simulink model "WM_Sim"  (R2013a)
settings: Solver=VariableStepDiscrete  StartTime=0.0  StopTime=WM.Sim.Time_length  RelTol=1e-3
InitFcn:
  | %if (matlab_sim)==false
  | 
  | %WM_Sim_config_smlnk_standalone;
  | 
  | %end
  | if isfield(WM.Sim,'BER_results')
  | WM.Sim = rmfield(WM.Sim,{'BER_results'});
  | end
  | if isfield(WM.Sim,'Uncoded_BER_results')
  | WM.Sim = rmfield(WM.Sim,{'Uncoded_BER_results'});
  | end
StopFcn:
  | if (matlab_sim)==false
  | WM.Sim.BER_results=BER_results_simout;
  | WM.Sim.Uncoded_BER_results=Uncoded_BER_results_simout;
  | %save_data_n_params(WM);
  | end
libraries: dspstat3 x15, dspmathops x8, dspsigops x3, dspsrcs4 x3, commdigbbndpm3 x3, commsink2 x2, commsynccomp2 x2, dspvision x2, commrandsrc2 x2, dspmtrx3 x2, commfilt2 x2, commchan3 x1
settings Model: Creator=leonardo  LastModifiedBy=leonardo
settings DataIOCC: SaveOutput=off  SignalLogging=off  DSMLogging=off  SaveTime=off
settings OptimizationCC: InlineParams=on  MemcpyThreshold=512
settings GRTTargetCC: CodeReplacementLibrary=C89/C90 (ANSI)

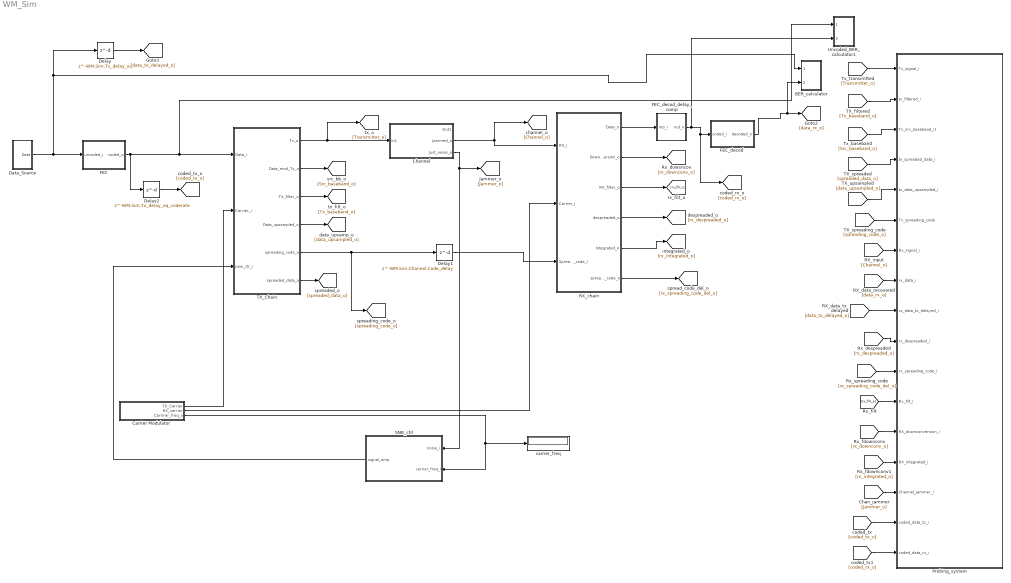
== system WM_Sim ==
  BER_calculator : Subsystem
  Carrier Modulator : Subsystem
  Channel : Subsystem
  Data_Source : Subsystem
  Delay : Delay  DelayLength=WM.Sim.Tx_delay_eq  InputProcessing=Columns as channels (frame based)
  Delay1 : Delay  DelayLength=WM.Sim.Channel.Code_delay  InputProcessing=Columns as channels (frame based)
  Delay2 : Delay  DelayLength=WM.Sim.Tx_delay_eq_coderate  InputProcessing=Columns as channels (frame based)
  FEC : Subsystem
  FEC_decod : Subsystem
  FEC_decod_delay_comp : Subsystem
  Probing_system : Subsystem
  RX_chain : Subsystem
  SNR_ctrl : Subsystem
  TX_Chain : Subsystem
  Uncoded_BER_calculator1 : Subsystem
  carrier_freq : Display
  wires:
  Carrier Modulator/1(TX_Carrier) -> TX_Chain/2(Carrier_i)
  TX_Chain/1(Tx_o) -> Channel/1(In1), [Transmitter_o]
  [Transmitter_o] -> Probing_system/1(Tx_signal_i)
  [Channel_o] -> Probing_system/7(Rx_signal_i)
  [data_tx_delayed_o] -> Probing_system/9(rx_data_tx_delayed_i)
  [data_rx_o] -> Probing_system/8(rx_data_i)
  TX_Chain/5(spreading_code_o) -> [spreading_code_o], Delay1/1
  Delay1/1 -> RX_chain/3(Spreading_code_i)
  TX_Chain/3(TX_filter_o) -> [Tx_baseband_o]
  [Tx_baseband_o] -> Probing_system/2(tx_filtered_i)
  TX_Chain/2(Data_mod_Tx_o) -> [Src_baseband_o]
  [Src_baseband_o] -> Probing_system/3(Tx_src_baseband_i1)
  TX_Chain/6(spreaded_data_o) -> [spreaded_data_o]
  [spreaded_data_o] -> Probing_system/4(tx_spreaded_data_i)
  [data_upsampled_o] -> Probing_system/5(tx_data_upsampled_i)
  RX_chain/3(RX_filter_o) -> [rx_filt_o]
  RX_chain/4(despreaded_o) -> [rx_despreaded_o]
  [rx_despreaded_o] -> Probing_system/10(rx_despreaded_i)
  [rx_spreading_code_del_o] -> Probing_system/11(rx_spreading_code_i)
  [spreading_code_o] -> Probing_system/6(Tx_spreading_code)
  [rx_filt_o] -> Probing_system/12(Rx_filt_i)
  RX_chain/2(Downconversion_o) -> [rx_downconv_o]
  [rx_downconv_o] -> Probing_system/13(RX_downconversion_i)
  RX_chain/5(Integrated_o) -> [rx_integrated_o]
  [rx_integrated_o] -> Probing_system/14(RX_integrated_i)
  Channel/3(Just_noise_o) -> [Jammer_o], SNR_ctrl/1(noise_i)
  SNR_ctrl/1(signal_amp) -> TX_Chain/3(pow_ctr_i)
  [Jammer_o] -> Probing_system/15(Channel_jammer_i)
  RX_chain/6(spreading_code_o) -> [rx_spreading_code_del_o]
  Carrier Modulator/3(Carrirer_freq_o) -> SNR_ctrl/2(carrier_freq_i), carrier_freq/1
  Data_Source/1(Data) -> FEC/1(uncoded_i), BER_calculator/1(Tx_delayed_data_i), Delay/1
  FEC/1(coded_o) -> TX_Chain/1(Data_i), Uncoded_BER_calculator1/1(Tx_delayed_data_i), Delay2/1
  Channel/2(Jammed_o) -> [Channel_o], RX_chain/1(RX_i)
  FEC_decod/1(decoded_o) -> BER_calculator/2(Rx_data_i), [data_rx_o]
  Carrier Modulator/2(RX_carrier) -> RX_chain/2(Carrier_i)
  TX_Chain/4(Data_upsampled_o) -> [data_upsampled_o]
  Delay/1 -> [data_tx_delayed_o]
  [coded_tx_o] -> Probing_system/16(coded_data_tx_i)
  Delay2/1 -> [coded_tx_o]
  [coded_rx_o] -> Probing_system/17(coded_data_rx_i)
  FEC_decod_delay_comp/1(out_o) -> Uncoded_BER_calculator1/2(Rx_data_i), [coded_rx_o], FEC_decod/1(coded_i)
  RX_chain/1(Data_o) -> FEC_decod_delay_comp/1(inp_i)

== system WM_Sim/BER_calculator ==
  Tx_delayed_data_i : Inport
  Rx_data_i : Inport  Port=2
  Display : Display
  Error Rate Calculation : commsink2/Error Rate Calculation  N=WM.Sim.Tx_delay_eq  st_delay=WM.Sim.Frame_len  cp_mode=Entire frame  subframe=[]  PMode=Port  WsName=ErrorVec  RsMode2=off  stop=off  numErr=100  maxBits=1e6
  To Workspace : ToWorkspace  VariableName=BER_results_simout  SampleTime=-1  SaveFormat=Timeseries
  wires:
  Rx_data_i/1 -> Error Rate Calculation/2
  Tx_delayed_data_i/1 -> Error Rate Calculation/1
  Error Rate Calculation/1 -> To Workspace/1, Display/1

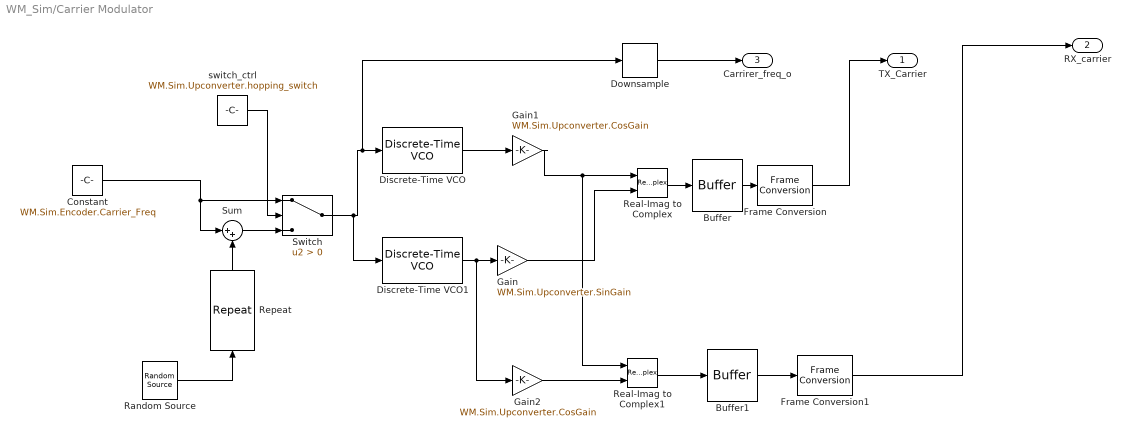
== system WM_Sim/Carrier Modulator ==
  Buffer : Buffer  N=int32(WM.Sim.Frame_len)  TreatMby1Signals=One channel
  Buffer1 : Buffer  N=int32(WM.Sim.Frame_len)  TreatMby1Signals=One channel
  Constant : Constant  Value=WM.Sim.Encoder.Carrier_Freq  VectorParams1D=off
  Discrete-Time VCO : commsynccomp2/Discrete-Time VCO  Ac=1  Fc=0  Kc=1  Ph=0  ts=WM.Sim.SampleTimes.Tchannel
  Discrete-Time VCO1 : commsynccomp2/Discrete-Time VCO  Ac=1  Fc=0  Kc=1  Ph=pi/4  ts=WM.Sim.SampleTimes.Tchannel
  Downsample : dspsigops/Downsample  N=int32(WM.Sim.Frame_len)  phase=0  InputProcessing=Columns as channels (frame based)  RateOptions=Allow multirate processing  smode=Allow multirate  fmode=Maintain input frame size  ic=0
  Frame Conversion : FrameConversion
  Frame Conversion1 : FrameConversion
  Gain : Gain  Gain=WM.Sim.Upconverter.SinGain
  Gain1 : Gain  Gain=WM.Sim.Upconverter.CosGain
  Gain2 : Gain  Gain=WM.Sim.Upconverter.CosGain
  Random Source : dspsrcs4/Random Source  SrcType=Uniform  NormMethod=Ziggurat  CltLength=12  MinVal=-WM.Sim.Upconverter.hopping_band/2  MaxVal=+WM.Sim.Upconverter.hopping_band/2  MeanVal=0  VarVal=1  RepMode=Specify seed  rawSeed=WM.Sim.Upconverter.Seed_hopping  IsInherit=off  SampMode=Discrete  SampTime=WM.Sim.SampleTimes.Tchannel*WM.Sim.Upconverter.hopping_div_vact  SampFrame=1  DataType=Double  OutComplex=Real
  Real-Imag to Complex : RealImagToComplex
  Real-Imag to Complex1 : RealImagToComplex
  Repeat : dspsigops/Repeat  N=WM.Sim.Upconverter.hopping_div_vact  InputProcessing=Columns as channels (frame based)  RateOptions=Allow multirate processing  ic=0  mode=Unused parameter value
  Sum : Sum  Inputs=|++
  Switch : Switch  Criteria=u2 > Threshold
  switch_ctrl : Constant  Value=WM.Sim.Upconverter.hopping_switch
  TX_Carrier : Outport
  RX_carrier : Outport  Port=2
  Carrirer_freq_o : Outport  Port=3
  wires:
  Buffer/1 -> Frame Conversion/1
  Gain/1 -> Real-Imag to Complex/2
  Buffer1/1 -> Frame Conversion1/1
  Constant/1 -> Switch/1, Sum/1
  Frame Conversion/1 -> TX_Carrier/1
  Discrete-Time VCO1/1 -> Gain2/1, Gain/1
  Real-Imag to Complex1/1 -> Buffer1/1
  Frame Conversion1/1 -> RX_carrier/1
  Discrete-Time VCO/1 -> Gain1/1
  Gain1/1 -> Real-Imag to Complex1/1, Real-Imag to Complex/1
  Gain2/1 -> Real-Imag to Complex1/2
  Real-Imag to Complex/1 -> Buffer/1
  Random Source/1 -> Repeat/1
  Sum/1 -> Switch/3
  Switch/1 -> Discrete-Time VCO1/1, Downsample/1, Discrete-Time VCO/1
  switch_ctrl/1 -> Switch/2
  Repeat/1 -> Sum/2
  Downsample/1 -> Carrirer_freq_o/1

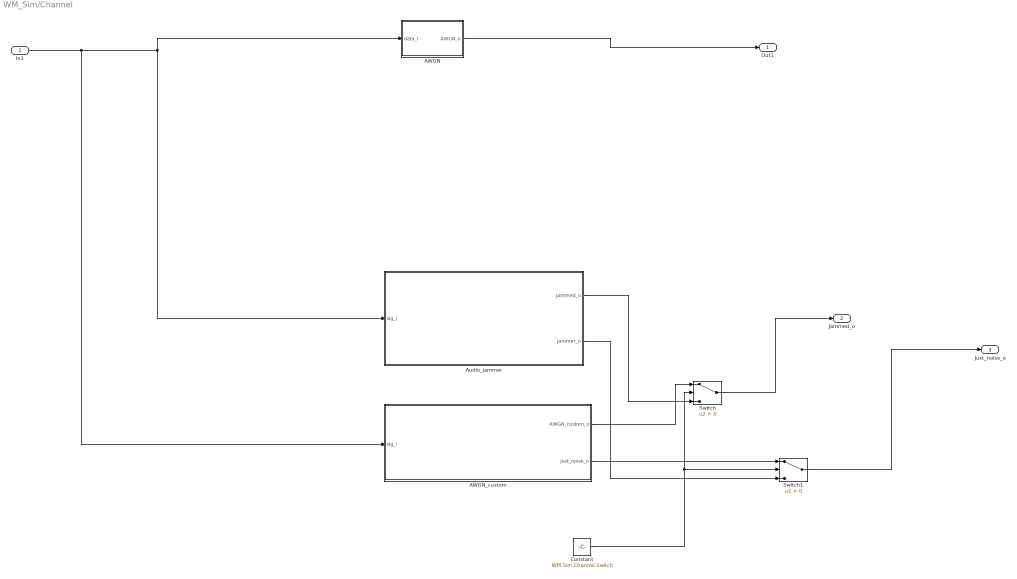
== system WM_Sim/Channel ==
  In1 : Inport
  AWGN : Subsystem
  AWGN_custom : Subsystem
  Audio_jammer : Subsystem
  Constant : Constant  Value=WM.Sim.Channel.Switch  SampleTime=WM.Sim.Frame_len/WM.Sim.Fs_audio
  Switch : Switch  Criteria=u2 > Threshold
  Switch1 : Switch  Criteria=u2 > Threshold
  Out1 : Outport
  Jammed_o : Outport  Port=2
  Just_noise_o : Outport  Port=3
  wires:
  In1/1 -> AWGN_custom/1(sig_i), Audio_jammer/1(sig_i), AWGN/1(data_i)
  AWGN/1(AWGN_o) -> Out1/1
  Constant/1 -> Switch1/2, Switch/2
  AWGN_custom/1(AWGN_custom_o) -> Switch/1
  Switch/1 -> Jammed_o/1
  Switch1/1 -> Just_noise_o/1
  AWGN_custom/2(just_noise_o) -> Switch1/1
  Audio_jammer/1(Jammed_o) -> Switch/3
  Audio_jammer/2(jammer_o) -> Switch1/3

== system WM_Sim/Data_Source ==
  Buffer : Buffer  N=WM.Sim.Frame_len  TreatMby1Signals=One channel
  Constant : Constant  VectorParams1D=off  SampleTime=WM.Sim.SampleTimes.Tsource  FramePeriod=WM.Sim.SampleTimes.Tsource
  Constant1 : Constant  Value=WM.Sim.Encoder.Source.Switch  VectorParams1D=off  FramePeriod=WM.Sim.SampleTimes.Tspreader
  Frame Conversion : FrameConversion
  Random Integer Generator : commrandsrc2/Random Integer Generator  mul=WM.Sim.order_M  seed=WM.Sim.seed_rand_msg  Ts=WM.Sim.SampleTimes.Tsource  frameBased=on  sampPerFrame=WM.Sim.Frame_len  orient=off  outDataType=double
  Switch : Switch  Criteria=u2 > Threshold
  Data : Outport
  wires:
  Random Integer Generator/1 -> Switch/1
  Constant/1 -> Buffer/1
  Buffer/1 -> Frame Conversion/1
  Frame Conversion/1 -> Switch/3
  Constant1/1 -> Switch/2
  Switch/1 -> Data/1

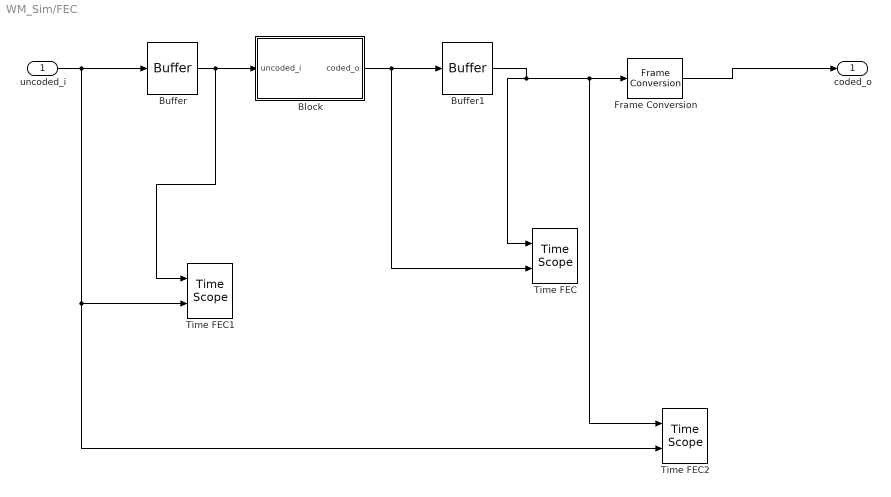
== system WM_Sim/FEC ==
  uncoded_i : Inport
  Block : Subsystem
  Buffer : Buffer  N=WM.Sim.Message_length  TreatMby1Signals=One channel
  Buffer1 : Buffer  N=WM.Sim.Frame_len  TreatMby1Signals=One channel
  Frame Conversion : FrameConversion
  Time FEC : TimeScope  NumInputPorts=2  DefaultConfigurationName=spbscopes.TimeScopeBlockCfg
      settings: CopyFcn=scopeextensions.ScopeBlock.callback(gcbh, 'onBlockCopy', gcbh);  DeleteFcn=scopeextensions.ScopeBlock.callback(gcbh, 'onBlockDelete');  PreSaveFcn=scopeextensions.ScopeBlock.callback(gcbh, 'onModelSave');  NameChangeFcn=scopeextensions.ScopeBlock.callback(gcbh, 'onBlockRename');  CloseFcn=scopeextensions.ScopeBlock.callback(gcbh, 'onBlockClose');  PreDeleteFcn=scopeextensions.ScopeBlock.callback(gcbh, 'onBlockPreDelete');
  Time FEC1 : TimeScope  NumInputPorts=2  DefaultConfigurationName=spbscopes.TimeScopeBlockCfg
      settings: CopyFcn=scopeextensions.ScopeBlock.callback(gcbh, 'onBlockCopy', gcbh);  DeleteFcn=scopeextensions.ScopeBlock.callback(gcbh, 'onBlockDelete');  PreSaveFcn=scopeextensions.ScopeBlock.callback(gcbh, 'onModelSave');  NameChangeFcn=scopeextensions.ScopeBlock.callback(gcbh, 'onBlockRename');  CloseFcn=scopeextensions.ScopeBlock.callback(gcbh, 'onBlockClose');  PreDeleteFcn=scopeextensions.ScopeBlock.callback(gcbh, 'onBlockPreDelete');
  Time FEC2 : TimeScope  NumInputPorts=2  DefaultConfigurationName=spbscopes.TimeScopeBlockCfg
      settings: CopyFcn=scopeextensions.ScopeBlock.callback(gcbh, 'onBlockCopy', gcbh);  DeleteFcn=scopeextensions.ScopeBlock.callback(gcbh, 'onBlockDelete');  PreSaveFcn=scopeextensions.ScopeBlock.callback(gcbh, 'onModelSave');  NameChangeFcn=scopeextensions.ScopeBlock.callback(gcbh, 'onBlockRename');  CloseFcn=scopeextensions.ScopeBlock.callback(gcbh, 'onBlockClose');  PreDeleteFcn=scopeextensions.ScopeBlock.callback(gcbh, 'onBlockPreDelete');
  coded_o : Outport
  wires:
  uncoded_i/1 -> Time FEC2/2, Time FEC1/2, Buffer/1
  Frame Conversion/1 -> coded_o/1
  Block/1(coded_o) -> Time FEC/2, Buffer1/1
  Buffer1/1 -> Time FEC/1, Time FEC2/1, Frame Conversion/1
  Buffer/1 -> Time FEC1/1, Block/1(uncoded_i)

== system WM_Sim/FEC_decod ==
  coded_i : Inport
  Block : Subsystem
  Buffer : Buffer  N=WM.Sim.Codeword_length  TreatMby1Signals=One channel
  Frame Conversion : FrameConversion
  Time FEC_decod : TimeScope  NumInputPorts=2  DefaultConfigurationName=spbscopes.TimeScopeBlockCfg
      settings: CopyFcn=scopeextensions.ScopeBlock.callback(gcbh, 'onBlockCopy', gcbh);  DeleteFcn=scopeextensions.ScopeBlock.callback(gcbh, 'onBlockDelete');  PreSaveFcn=scopeextensions.ScopeBlock.callback(gcbh, 'onModelSave');  NameChangeFcn=scopeextensions.ScopeBlock.callback(gcbh, 'onBlockRename');  CloseFcn=scopeextensions.ScopeBlock.callback(gcbh, 'onBlockClose');  PreDeleteFcn=scopeextensions.ScopeBlock.callback(gcbh, 'onBlockPreDelete');
  Time FEC_decod1 : TimeScope  NumInputPorts=2  DefaultConfigurationName=spbscopes.TimeScopeBlockCfg
      settings: CopyFcn=scopeextensions.ScopeBlock.callback(gcbh, 'onBlockCopy', gcbh);  DeleteFcn=scopeextensions.ScopeBlock.callback(gcbh, 'onBlockDelete');  PreSaveFcn=scopeextensions.ScopeBlock.callback(gcbh, 'onModelSave');  NameChangeFcn=scopeextensions.ScopeBlock.callback(gcbh, 'onBlockRename');  CloseFcn=scopeextensions.ScopeBlock.callback(gcbh, 'onBlockClose');  PreDeleteFcn=scopeextensions.ScopeBlock.callback(gcbh, 'onBlockPreDelete');
  Unbuff : Subsystem
  decoded_o : Outport
  wires:
  coded_i/1 -> Time FEC_decod1/2, Buffer/1
  Frame Conversion/1 -> decoded_o/1
  Buffer/1 -> Time FEC_decod1/1, Block/1(coded_i)
  Block/1(decoded_o) -> Time FEC_decod/2, Unbuff/1(buffered_i)
  Unbuff/1(unbuffered_o) -> Time FEC_decod/1, Frame Conversion/1

== system WM_Sim/FEC_decod_delay_comp ==
  inp_i : Inport
  out_o : Outport
  wires:
  inp_i/1 -> out_o/1

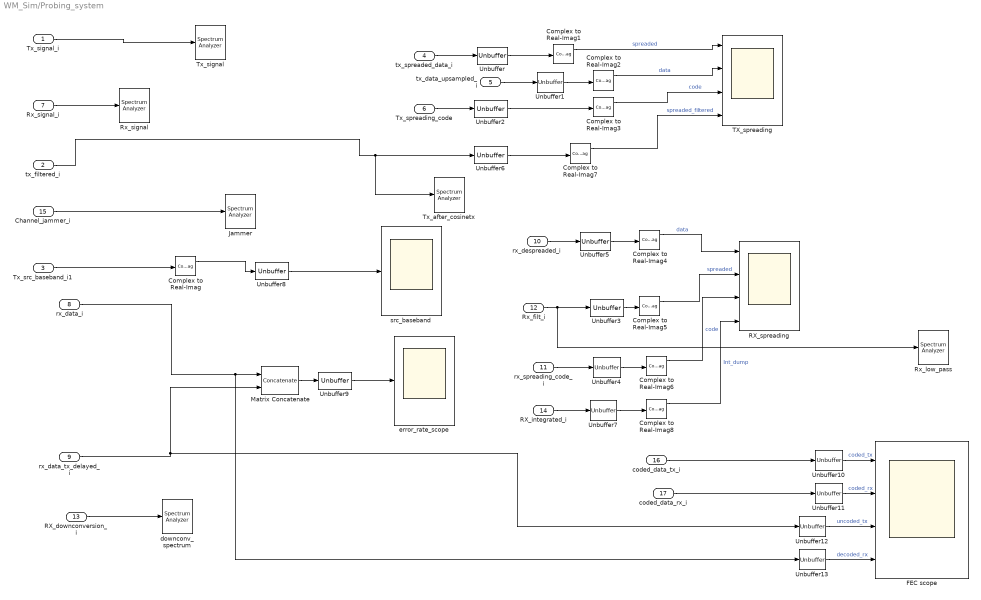
== system WM_Sim/Probing_system ==
  Tx_signal_i : Inport
  tx_filtered_i : Inport  Port=2
  Tx_src_baseband_i1 : Inport  Port=3
  tx_spreaded_data_i : Inport  Port=4
  tx_data_upsampled_i : Inport  Port=5
  Tx_spreading_code : Inport  Port=6
  Rx_signal_i : Inport  Port=7
  rx_data_i : Inport  Port=8
  rx_data_tx_delayed_i : Inport  Port=9
  rx_despreaded_i : Inport  Port=10
  rx_spreading_code_i : Inport  Port=11
  Rx_filt_i : Inport  Port=12
  RX_downconversion_i : Inport  Port=13
  RX_integrated_i : Inport  Port=14
  Channel_jammer_i : Inport  Port=15
  coded_data_tx_i : Inport  Port=16
  coded_data_rx_i : Inport  Port=17
  Complex to Real-Imag{,1..8} (9 alike) : ComplexToRealImag
  FEC scope : Scope  NumInputPorts=4
      settings: YMin=-5~-5~-5~-5  YMax=5~5~5~5  SaveName=ScopeData6
  Jammer : SpectrumAnalyzer
      settings: CopyFcn=scopeextensions.ScopeBlock.callback(gcbh, 'onBlockCopy', gcbh);  DeleteFcn=scopeextensions.ScopeBlock.callback(gcbh, 'onBlockDelete');  PreSaveFcn=scopeextensions.ScopeBlock.callback(gcbh, 'onModelSave');  NameChangeFcn=scopeextensions.ScopeBlock.callback(gcbh, 'onBlockRename');  CloseFcn=scopeextensions.ScopeBlock.callback(gcbh, 'onBlockClose');  PreDeleteFcn=scopeextensions.ScopeBlock.callback(gcbh, 'onBlockPreDelete');
  Matrix Concatenate : Concatenate  Mode=Multidimensional array  ConcatenateDimension=2
  RX_spreading : Scope  NumInputPorts=4
      settings: YMin=-0.0225~-0.025~-1~-1000  YMax=0.02~0.025~1~1750  SaveName=ScopeData3  MaxDataPoints=WM.Sim.Probe_system.RX_spreading.data_history_len
  Rx_low_pass : SpectrumAnalyzer
      settings: CopyFcn=scopeextensions.ScopeBlock.callback(gcbh, 'onBlockCopy', gcbh);  DeleteFcn=scopeextensions.ScopeBlock.callback(gcbh, 'onBlockDelete');  PreSaveFcn=scopeextensions.ScopeBlock.callback(gcbh, 'onModelSave');  NameChangeFcn=scopeextensions.ScopeBlock.callback(gcbh, 'onBlockRename');  CloseFcn=scopeextensions.ScopeBlock.callback(gcbh, 'onBlockClose');  PreDeleteFcn=scopeextensions.ScopeBlock.callback(gcbh, 'onBlockPreDelete');
  Rx_signal : SpectrumAnalyzer
      settings: CopyFcn=scopeextensions.ScopeBlock.callback(gcbh, 'onBlockCopy', gcbh);  DeleteFcn=scopeextensions.ScopeBlock.callback(gcbh, 'onBlockDelete');  PreSaveFcn=scopeextensions.ScopeBlock.callback(gcbh, 'onModelSave');  NameChangeFcn=scopeextensions.ScopeBlock.callback(gcbh, 'onBlockRename');  CloseFcn=scopeextensions.ScopeBlock.callback(gcbh, 'onBlockClose');  PreDeleteFcn=scopeextensions.ScopeBlock.callback(gcbh, 'onBlockPreDelete');
  TX_spreading : Scope  NumInputPorts=4
      settings: YMin=-5~-5~-5~-5  YMax=5~5~5~5  SaveName=ScopeData2
  Tx_after_cosinetx : SpectrumAnalyzer
      settings: CopyFcn=scopeextensions.ScopeBlock.callback(gcbh, 'onBlockCopy', gcbh);  DeleteFcn=scopeextensions.ScopeBlock.callback(gcbh, 'onBlockDelete');  PreSaveFcn=scopeextensions.ScopeBlock.callback(gcbh, 'onModelSave');  NameChangeFcn=scopeextensions.ScopeBlock.callback(gcbh, 'onBlockRename');  CloseFcn=scopeextensions.ScopeBlock.callback(gcbh, 'onBlockClose');  PreDeleteFcn=scopeextensions.ScopeBlock.callback(gcbh, 'onBlockPreDelete');
  Tx_signal : SpectrumAnalyzer
      settings: CopyFcn=scopeextensions.ScopeBlock.callback(gcbh, 'onBlockCopy', gcbh);  DeleteFcn=scopeextensions.ScopeBlock.callback(gcbh, 'onBlockDelete');  PreSaveFcn=scopeextensions.ScopeBlock.callback(gcbh, 'onModelSave');  NameChangeFcn=scopeextensions.ScopeBlock.callback(gcbh, 'onBlockRename');  CloseFcn=scopeextensions.ScopeBlock.callback(gcbh, 'onBlockClose');  PreDeleteFcn=scopeextensions.ScopeBlock.callback(gcbh, 'onBlockPreDelete');
  Unbuffer{,1..13} (14 alike) : Unbuffer  SampleBasedProcessing=Same as frame based
  downconv_spectrum : SpectrumAnalyzer
      settings: CopyFcn=scopeextensions.ScopeBlock.callback(gcbh, 'onBlockCopy', gcbh);  DeleteFcn=scopeextensions.ScopeBlock.callback(gcbh, 'onBlockDelete');  PreSaveFcn=scopeextensions.ScopeBlock.callback(gcbh, 'onModelSave');  NameChangeFcn=scopeextensions.ScopeBlock.callback(gcbh, 'onBlockRename');  CloseFcn=scopeextensions.ScopeBlock.callback(gcbh, 'onBlockClose');  PreDeleteFcn=scopeextensions.ScopeBlock.callback(gcbh, 'onBlockPreDelete');
  error_rate_scope : Scope
  src_baseband : Scope
  wires:
  Rx_signal_i/1 -> Rx_signal/1
  Matrix Concatenate/1 -> Unbuffer9/1
  rx_data_tx_delayed_i/1 -> Unbuffer12/1, Matrix Concatenate/2
  rx_data_i/1 -> Unbuffer13/1, Matrix Concatenate/1
  tx_filtered_i/1 -> Tx_after_cosinetx/1, Unbuffer6/1
  Tx_src_baseband_i1/1 -> Complex to Real-Imag/1
  Complex to Real-Imag/1 -> Unbuffer8/1
  tx_data_upsampled_i/1 -> Unbuffer1/1
  tx_spreaded_data_i/1 -> Unbuffer/1
  Tx_spreading_code/1 -> Unbuffer2/1
  Complex to Real-Imag1/1 -> TX_spreading/1  "spreaded"
  Unbuffer/1 -> Complex to Real-Imag1/1
  Unbuffer1/1 -> Complex to Real-Imag2/1
  Unbuffer2/1 -> Complex to Real-Imag3/1
  Complex to Real-Imag2/1 -> TX_spreading/2  "data"
  Complex to Real-Imag3/1 -> TX_spreading/3  "code"
  rx_despreaded_i/1 -> Unbuffer5/1
  rx_spreading_code_i/1 -> Unbuffer4/1
  Rx_filt_i/1 -> Rx_low_pass/1, Unbuffer3/1
  Unbuffer5/1 -> Complex to Real-Imag4/1
  Unbuffer3/1 -> Complex to Real-Imag5/1
  Unbuffer4/1 -> Complex to Real-Imag6/1
  Complex to Real-Imag4/1 -> RX_spreading/1  "data"
  Complex to Real-Imag5/1 -> RX_spreading/2  "spreaded"
  Complex to Real-Imag6/1 -> RX_spreading/3  "code"
  Complex to Real-Imag7/1 -> TX_spreading/4  "spreaded_filtered"
  Unbuffer6/1 -> Complex to Real-Imag7/1
  RX_integrated_i/1 -> Unbuffer7/1
  Unbuffer7/1 -> Complex to Real-Imag8/1
  Complex to Real-Imag8/1 -> RX_spreading/4  "Int_dump"
  Channel_jammer_i/1 -> Jammer/1
  Tx_signal_i/1 -> Tx_signal/1
  RX_downconversion_i/1 -> downconv_spectrum/1
  Unbuffer8/1 -> src_baseband/1
  Unbuffer9/1 -> error_rate_scope/1
  Unbuffer12/1 -> FEC scope/3  "uncoded_tx"
  Unbuffer10/1 -> FEC scope/1  "coded_tx"
  Unbuffer13/1 -> FEC scope/4  "decoded_rx"
  Unbuffer11/1 -> FEC scope/2  "coded_rx"
  coded_data_tx_i/1 -> Unbuffer10/1
  coded_data_rx_i/1 -> Unbuffer11/1

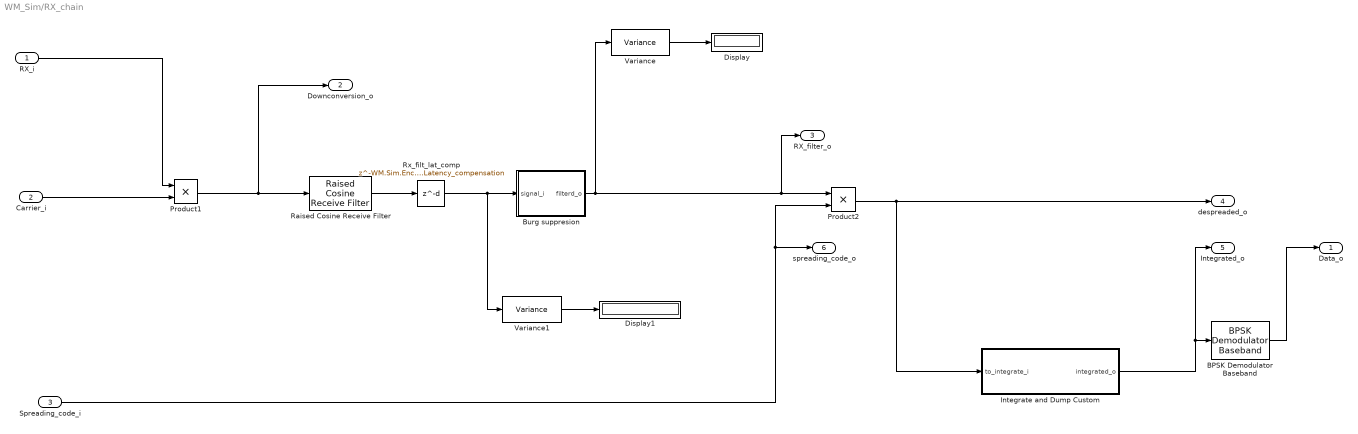
== system WM_Sim/RX_chain ==
  RX_i : Inport
  Carrier_i : Inport  Port=2
  Spreading_code_i : Inport  Port=3
  BPSK Demodulator Baseband : commdigbbndpm3/BPSK Demodulator Baseband  Ph=0  DecType=Hard decision  VarSource=Dialog  Variance=1  outDtype=Inherit via internal rule  derotateFactorWordLen=16
  Burg suppresion : Subsystem
  Display : Display
  Display1 : Display
  Integrate and Dump Custom : Subsystem
  Product1 : Product
  Product2 : Product
  Raised Cosine Receive Filter : commfilt2/Raised Cosine Receive Filter  filtType=Normal  N=WM.Sim.Encoder.TxFilter.OversamplingFactor  D=(2*(WM.Sim.Encoder.TxFilter.GroupDelay))/2  R=WM.Sim.Encoder.TxFilter.RollOffFactor  sampMode=Mute  saveAsFlag=0  rateMode=Downsampling  downFactor=WM.Sim.Encoder.TxFilter.OversamplingFactor  downOffset=0  framing=Allow multirate processing  InputProcessing=Columns as channels (frame based)  checkGain=User-specified  filterGain=1  checkCoeff=on  variableName=hRxFilt  launchFVT=off  roundingMode=Floor  overflowMode=off
  Rx_filt_lat_comp : Delay  DelayLength=WM.Sim.Encoder.TxFilter.Latency_compensation  InputProcessing=Columns as channels (frame based)
  Variance : dspstat3/Variance  run=on  reset_popup=None  InputProcessing=Columns as channels (frame based)  directionMode=Each column  dimension=1  treatSBRowAsCol=on  roiEnable=off  roiType=Rectangles  roiPortion=Entire ROI  roiOutput=Individual statistics for each ROI  roiFlag=off  roundingMode=Floor  overflowMode=off
  Variance1 : dspstat3/Variance  run=on  reset_popup=None  InputProcessing=Columns as channels (frame based)  directionMode=Each column  dimension=1  treatSBRowAsCol=on  roiEnable=off  roiType=Rectangles  roiPortion=Entire ROI  roiOutput=Individual statistics for each ROI  roiFlag=off  roundingMode=Floor  overflowMode=off
  Data_o : Outport
  Downconversion_o : Outport  Port=2
  RX_filter_o : Outport  Port=3
  despreaded_o : Outport  Port=4
  Integrated_o : Outport  Port=5
  spreading_code_o : Outport  Port=6
  wires:
  BPSK Demodulator Baseband/1 -> Data_o/1
  Product1/1 -> Raised Cosine Receive Filter/1, Downconversion_o/1
  Raised Cosine Receive Filter/1 -> Rx_filt_lat_comp/1
  RX_i/1 -> Product1/1
  Carrier_i/1 -> Product1/2
  Integrate and Dump Custom/1(integrated_o) -> Integrated_o/1, BPSK Demodulator Baseband/1
  Product2/1 -> Integrate and Dump Custom/1(to_integrate_i), despreaded_o/1
  Burg suppresion/1(filterd_o) -> Variance/1, RX_filter_o/1, Product2/1
  Rx_filt_lat_comp/1 -> Burg suppresion/1(signal_i), Variance1/1
  Spreading_code_i/1 -> spreading_code_o/1, Product2/2
  Variance/1 -> Display/1
  Variance1/1 -> Display1/1

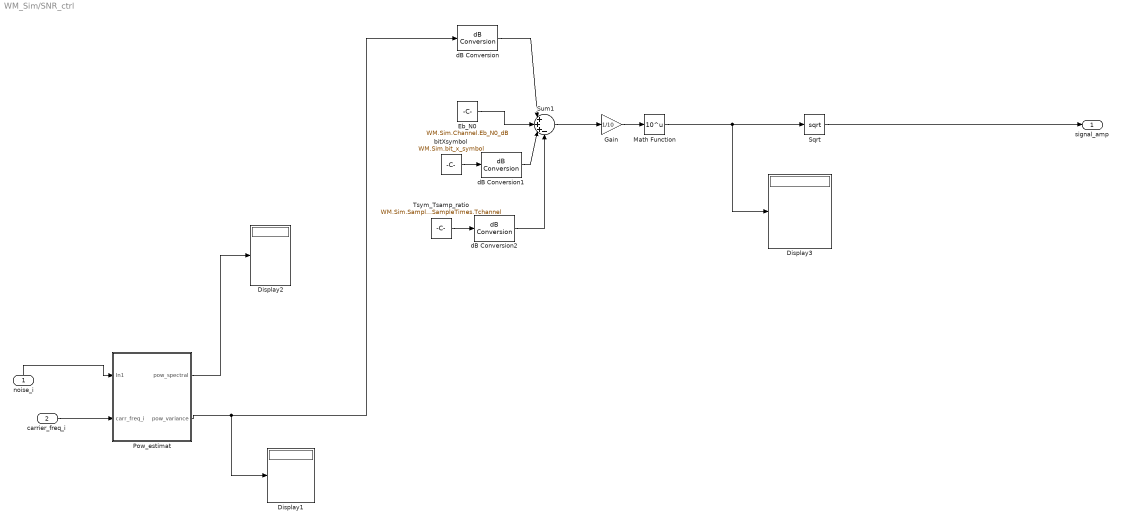
== system WM_Sim/SNR_ctrl ==
  noise_i : Inport
  carrier_freq_i : Inport  Port=2
  Display1 : Display
  Display2 : Display
  Display3 : Display
  Eb_N0 : Constant  Value=WM.Sim.Channel.Eb_N0_dB
  Gain : Gain  Gain=1/10
  Math Function : Math  Operator=10^u  SaturateOnIntegerOverflow=on
  Pow_estimat : Subsystem
  Sqrt : Sqrt  SaturateOnIntegerOverflow=on
  Sum1 : Sum  Inputs=|+++-
  Tsym_Tsamp_ratio : Constant  Value=WM.Sim.SampleTimes.Tcoded/WM.Sim.SampleTimes.Tchannel
      settings: SamplingMode=Frame based
  bitXsymbol : Constant  Value=WM.Sim.bit_x_symbol
  dB Conversion : dspmathops/dB Conversion  dBtype=dB  intype=Power  R=1  fuzz=off
  dB Conversion1 : dspmathops/dB Conversion  dBtype=dB  intype=Power  R=1  fuzz=off
  dB Conversion2 : dspmathops/dB Conversion  dBtype=dB  intype=Power  R=1  fuzz=off
  signal_amp : Outport
  wires:
  Sum1/1 -> Gain/1
  Eb_N0/1 -> Sum1/2
  Tsym_Tsamp_ratio/1 -> dB Conversion2/1
  dB Conversion/1 -> Sum1/1
  dB Conversion2/1 -> Sum1/4
  bitXsymbol/1 -> dB Conversion1/1
  dB Conversion1/1 -> Sum1/3
  Gain/1 -> Math Function/1
  Math Function/1 -> Display3/1, Sqrt/1
  Sqrt/1 -> signal_amp/1
  Pow_estimat/2(pow_variance) -> Display1/1, dB Conversion/1
  noise_i/1 -> Pow_estimat/1(In1)
  Pow_estimat/1(pow_spectral) -> Display2/1
  carrier_freq_i/1 -> Pow_estimat/2(carr_freq_i)

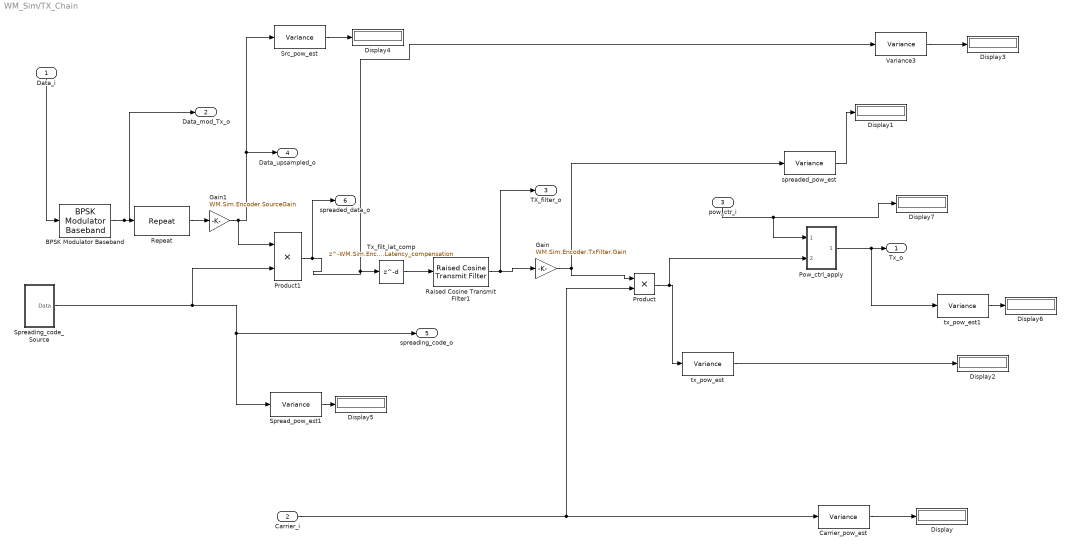
== system WM_Sim/TX_Chain ==
  Data_i : Inport
  Carrier_i : Inport  Port=2
  pow_ctr_i : Inport  Port=3
  BPSK Modulator Baseband : commdigbbndpm3/BPSK Modulator Baseband  Ph=0  outDtype=double  outWordLen=16  outUDDataType=sfix(16)  outFracLenMode=Best precision  outFracLen=15
  Carrier_pow_est : dspstat3/Variance  run=on  reset_popup=None  InputProcessing=Columns as channels (frame based)  directionMode=Each column  dimension=1  treatSBRowAsCol=on  roiEnable=off  roiType=Rectangles  roiPortion=Entire ROI  roiOutput=Individual statistics for each ROI  roiFlag=off  roundingMode=Floor  overflowMode=off
  Display{,1..7} (8 alike) : Display
  Gain : Gain  Gain=WM.Sim.Encoder.TxFilter.Gain
  Gain1 : Gain  Gain=WM.Sim.Encoder.SourceGain
  Pow_ctrl_apply : Subsystem
  Product : Product
  Product1 : Product
  Raised Cosine Transmit Filter1 : commfilt2/Raised Cosine Transmit Filter  filtType=Normal  D=(2*(WM.Sim.Encoder.TxFilter.GroupDelay))/2  R=WM.Sim.Encoder.TxFilter.RollOffFactor  sampMode=Mute  saveAsFlag=0  N=WM.Sim.Encoder.TxFilter.OversamplingFactor  framing=Allow multirate processing  InputProcessing=Columns as channels (frame based)  checkGain=Normalized  filterGain=1  checkCoeff=off  variableName=rcTxFilt1  launchFVT=off  roundingMode=Floor  overflowMode=off
  Repeat : dspsigops/Repeat  N=WM.Sim.Encoder.SF  InputProcessing=Columns as channels (frame based)  RateOptions=Allow multirate processing  ic=0  mode=Unused parameter value
  Spread_pow_est1 : dspstat3/Variance  run=on  reset_popup=None  InputProcessing=Columns as channels (frame based)  directionMode=Each column  dimension=1  treatSBRowAsCol=on  roiEnable=off  roiType=Rectangles  roiPortion=Entire ROI  roiOutput=Individual statistics for each ROI  roiFlag=off  roundingMode=Floor  overflowMode=off
  Spreading_code_Source : Subsystem
  Src_pow_est : dspstat3/Variance  run=on  reset_popup=None  InputProcessing=Columns as channels (frame based)  directionMode=Each column  dimension=1  treatSBRowAsCol=on  roiEnable=off  roiType=Rectangles  roiPortion=Entire ROI  roiOutput=Individual statistics for each ROI  roiFlag=off  roundingMode=Floor  overflowMode=off
  Tx_filt_lat_comp : Delay  DelayLength=WM.Sim.Encoder.TxFilter.Latency_compensation  InputProcessing=Columns as channels (frame based)
  Variance3 : dspstat3/Variance  run=on  reset_popup=None  InputProcessing=Columns as channels (frame based)  directionMode=Each column  dimension=1  treatSBRowAsCol=on  roiEnable=off  roiType=Rectangles  roiPortion=Entire ROI  roiOutput=Individual statistics for each ROI  roiFlag=off  roundingMode=Floor  overflowMode=off
  spreaded_pow_est : dspstat3/Variance  run=on  reset_popup=None  InputProcessing=Columns as channels (frame based)  directionMode=Each column  dimension=1  treatSBRowAsCol=on  roiEnable=off  roiType=Rectangles  roiPortion=Entire ROI  roiOutput=Individual statistics for each ROI  roiFlag=off  roundingMode=Floor  overflowMode=off
  tx_pow_est : dspstat3/Variance  run=on  reset_popup=None  InputProcessing=Columns as channels (frame based)  directionMode=Each column  dimension=1  treatSBRowAsCol=on  roiEnable=off  roiType=Rectangles  roiPortion=Entire ROI  roiOutput=Individual statistics for each ROI  roiFlag=off  roundingMode=Floor  overflowMode=off
  tx_pow_est1 : dspstat3/Variance  run=on  reset_popup=None  InputProcessing=Columns as channels (frame based)  directionMode=Each column  dimension=1  treatSBRowAsCol=on  roiEnable=off  roiType=Rectangles  roiPortion=Entire ROI  roiOutput=Individual statistics for each ROI  roiFlag=off  roundingMode=Floor  overflowMode=off
  Tx_o : Outport
  Data_mod_Tx_o : Outport  Port=2
  TX_filter_o : Outport  Port=3
  Data_upsampled_o : Outport  Port=4
  spreading_code_o : Outport  Port=5
  spreaded_data_o : Outport  Port=6
  wires:
  Data_i/1 -> BPSK Modulator Baseband/1
  BPSK Modulator Baseband/1 -> Data_mod_Tx_o/1, Repeat/1
  Product/1 -> Pow_ctrl_apply/2(data_i), tx_pow_est/1
  Gain/1 -> Product/1, spreaded_pow_est/1
  Carrier_pow_est/1 -> Display/1
  spreaded_pow_est/1 -> Display1/1
  Spreading_code_Source/1(Data) -> Spread_pow_est1/1, spreading_code_o/1, Product1/2
  Repeat/1 -> Gain1/1
  tx_pow_est/1 -> Display2/1
  Variance3/1 -> Display3/1
  Gain1/1 -> Product1/1, Data_upsampled_o/1, Src_pow_est/1
  Src_pow_est/1 -> Display4/1
  Spread_pow_est1/1 -> Display5/1
  Product1/1 -> spreaded_data_o/1, Tx_filt_lat_comp/1, Variance3/1
  Pow_ctrl_apply/1(data_o) -> tx_pow_est1/1, Tx_o/1
  tx_pow_est1/1 -> Display6/1
  pow_ctr_i/1 -> Pow_ctrl_apply/1(ctrl_pow_i), Display7/1
  Carrier_i/1 -> Carrier_pow_est/1, Product/2
  Tx_filt_lat_comp/1 -> Raised Cosine Transmit Filter1/1
  Raised Cosine Transmit Filter1/1 -> TX_filter_o/1, Gain/1

== system WM_Sim/Uncoded_BER_calculator1 ==
  Tx_delayed_data_i : Inport
  Rx_data_i : Inport  Port=2
  Display : Display
  Error Rate Calculation : commsink2/Error Rate Calculation  N=WM.Sim.Tx_delay_eq_coderate  st_delay=WM.Sim.Frame_len  cp_mode=Entire frame  subframe=[]  PMode=Port  WsName=ErrorVec  RsMode2=off  stop=off  numErr=100  maxBits=1e6
  To Workspace : ToWorkspace  VariableName=Uncoded_BER_results_simout  SampleTime=-1  SaveFormat=Timeseries
  wires:
  Error Rate Calculation/1 -> Display/1, To Workspace/1
  Tx_delayed_data_i/1 -> Error Rate Calculation/1
  Rx_data_i/1 -> Error Rate Calculation/2

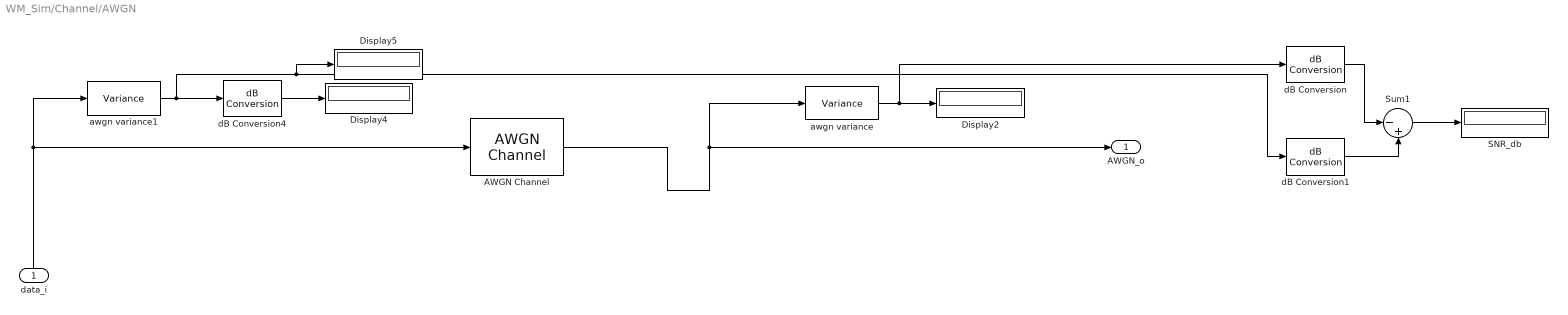
== system WM_Sim/Channel/AWGN ==
  data_i : Inport
  " awgn variance" : dspstat3/Variance  run=on  reset_popup=None  InputProcessing=Columns as channels (frame based)  directionMode=Each column  dimension=1  treatSBRowAsCol=on  roiEnable=off  roiType=Rectangles  roiPortion=Entire ROI  roiOutput=Individual statistics for each ROI  roiFlag=off  roundingMode=Floor  overflowMode=off
  " awgn variance1" : dspstat3/Variance  run=on  reset_popup=None  InputProcessing=Columns as channels (frame based)  directionMode=Each column  dimension=1  treatSBRowAsCol=on  roiEnable=off  roiType=Rectangles  roiPortion=Entire ROI  roiOutput=Individual statistics for each ROI  roiFlag=off  roundingMode=Floor  overflowMode=off
  AWGN Channel : commchan3/AWGN Channel  InputProcessing=Columns as channels (frame based)  seed=WM.Sim.Channel.AWGN_Custom.seed_noise_real  noiseMode="Signal to noise ratio  (Eb/No)"  EbNodB=WM.Sim.Channel.Eb_N0_dB  EsNodB=10  SNRdB=10  bitsPerSym=WM.Sim.bit_x_symbol  Ps=0.94  Tsym=WM.Sim.Encoder.Source_Ts  variance=1
  Display2 : Display
  Display4 : Display
  Display5 : Display
  SNR_db : Display
  Sum1 : Sum  Inputs=|-+
  dB Conversion : dspmathops/dB Conversion  dBtype=dB  intype=Power  R=1  fuzz=off
  dB Conversion1 : dspmathops/dB Conversion  dBtype=dB  intype=Power  R=1  fuzz=off
  dB Conversion4 : dspmathops/dB Conversion  dBtype=dB  intype=Power  R=1  fuzz=off
  AWGN_o : Outport
  wires:
  Sum1/1 -> SNR_db/1
  " awgn variance1"/1 -> Display5/1, dB Conversion1/1, dB Conversion4/1
  AWGN Channel/1 -> AWGN_o/1, " awgn variance"/1
  data_i/1 -> AWGN Channel/1, " awgn variance1"/1
  dB Conversion4/1 -> Display4/1
  dB Conversion1/1 -> Sum1/2
  dB Conversion/1 -> Sum1/1
  " awgn variance"/1 -> dB Conversion/1, Display2/1

== system WM_Sim/Channel/AWGN_custom ==
  sig_i : Inport
  AWGN Channel Custom : Subsystem
  Display1 : Display
  SNR_estimate : Subsystem
  custom awgn variance1 : dspstat3/Variance  run=on  reset_popup=None  InputProcessing=Columns as channels (frame based)  directionMode=Each column  dimension=1  treatSBRowAsCol=on  roiEnable=off  roiType=Rectangles  roiPortion=Entire ROI  roiOutput=Individual statistics for each ROI  roiFlag=off  roundingMode=Floor  overflowMode=off
  AWGN_custom_o : Outport
  just_noise_o : Outport  Port=2
  wires:
  sig_i/1 -> SNR_estimate/2(in_block_i), AWGN Channel Custom/1(data_i)
  custom awgn variance1/1 -> Display1/1
  AWGN Channel Custom/1(only_noise_o) -> just_noise_o/1
  AWGN Channel Custom/2(AWGN_o) -> SNR_estimate/1(out_block_i), AWGN_custom_o/1, custom awgn variance1/1

== system WM_Sim/Channel/Audio_jammer ==
  sig_i : Inport
  Audio_channel : Subsystem
  Complex to Real-Imag : ComplexToRealImag
  To Multimedia File : dspvision/To Multimedia File  outputFilename=./audio_test/jammed.wav  streamSelection=Audio only  videoCompressor=None (uncompressed)  audioCompressor=None (uncompressed)  imagePorts=Separate color signals  fileType=WAV  audioDatatype=16-bit integer  fourcc=RGB
  Jammed_o : Outport
  jammer_o : Outport  Port=2
  wires:
  Complex to Real-Imag/2 -> ?
  Audio_channel/1(mix_o) -> Jammed_o/1, Complex to Real-Imag/1
  sig_i/1 -> Audio_channel/1(data_i)
  Audio_channel/2(Jamm_o) -> jammer_o/1
  Complex to Real-Imag/1 -> To Multimedia File/1

== system WM_Sim/FEC/Block ==
  uncoded_i : Inport
  coded_o : Outport
  wires:
  uncoded_i/1 -> coded_o/1

== system WM_Sim/FEC_decod/Block ==
  coded_i : Inport
  decoded_o : Outport
  wires:
  coded_i/1 -> decoded_o/1

== system WM_Sim/FEC_decod/Unbuff ==
  buffered_i : Inport
  Buffer : Buffer  N=WM.Sim.Frame_len  TreatMby1Signals=One channel
  unbuffered_o : Outport
  wires:
  buffered_i/1 -> Buffer/1
  Buffer/1 -> unbuffered_o/1

== system WM_Sim/RX_chain/Burg suppresion ==
  signal_i : Inport
  filterd_o : Outport
  wires:
  signal_i/1 -> filterd_o/1

== system WM_Sim/RX_chain/Integrate and Dump Custom ==
  to_integrate_i : Inport
  Buffer : Buffer  N=WM.Sim.Encoder.SF
  Frame Conversion2 : FrameConversion
  Integrate and dumo : MATLAB Function  TreatAsAtomicUnit=on
  Transpose : dspmtrx3/Transpose  Hermitian=off  overflowFlag=off
  Transpose1 : dspmtrx3/Transpose  Hermitian=off  overflowFlag=off
  integrated_o : Outport
  wires:
  Transpose1/1 -> Frame Conversion2/1
  to_integrate_i/1 -> Transpose/1
  Transpose/1 -> Buffer/1
  Frame Conversion2/1 -> integrated_o/1
  Integrate and dumo/1(y) -> Transpose1/1
  Buffer/1 -> Integrate and dumo/1(u)

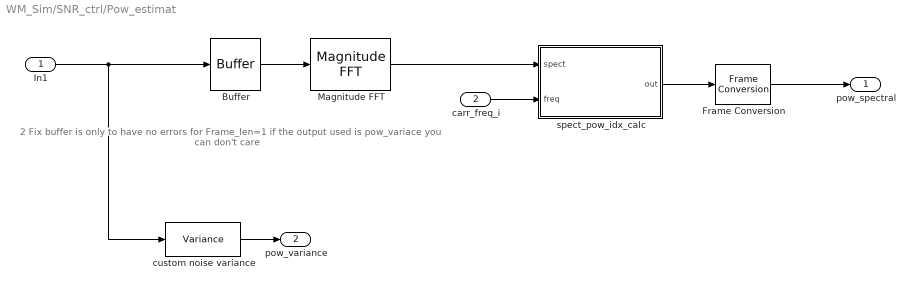
== system WM_Sim/SNR_ctrl/Pow_estimat ==
  note: 2 Fix buffer is only to have no errors for Frame_len=1
      | if the output used is pow_variace you can don't care
  In1 : Inport
  carr_freq_i : Inport  Port=2
  Buffer : Buffer  N=512  TreatMby1Signals=One channel
  Frame Conversion : FrameConversion
  Magnitude FFT : dspspect3/Magnitude FFT  mag_or_magsq=Magnitude squared  FFTImplementation=Auto  fftLenInherit=on  fftsize=256
  custom noise variance : dspstat3/Variance  run=on  reset_popup=None  InputProcessing=Columns as channels (frame based)  directionMode=Each column  dimension=1  treatSBRowAsCol=on  roiEnable=off  roiType=Rectangles  roiPortion=Entire ROI  roiOutput=Individual statistics for each ROI  roiFlag=off  roundingMode=Floor  overflowMode=off
  spect_pow_idx_calc : MATLAB Function  TreatAsAtomicUnit=on
  pow_spectral : Outport
  pow_variance : Outport  Port=2
  wires:
  In1/1 -> custom noise variance/1, Buffer/1
  custom noise variance/1 -> pow_variance/1
  Frame Conversion/1 -> pow_spectral/1
  carr_freq_i/1 -> spect_pow_idx_calc/2(freq)
  Magnitude FFT/1 -> spect_pow_idx_calc/1(spect)
  spect_pow_idx_calc/1(out) -> Frame Conversion/1
  Buffer/1 -> Magnitude FFT/1

== system WM_Sim/TX_Chain/Pow_ctrl_apply ==
  ctrl_pow_i : Inport
  data_i : Inport  Port=2
  Constant1 : Constant
  Constant2 : Constant  Value=WM.Sim.Encoder.Pow_ctrl.Switch
  Display8 : Display
  Product2 : Product  SampleTime=WM.Sim.Frame_len/WM.Sim.Fs_audio
  Switch : Switch  Criteria=u2 > Threshold
  data_o : Outport
  wires:
  Switch/1 -> Product2/1
  Constant1/1 -> Switch/3
  Constant2/1 -> Switch/2
  data_i/1 -> Product2/2
  Product2/1 -> data_o/1
  ctrl_pow_i/1 -> Switch/1, Display8/1

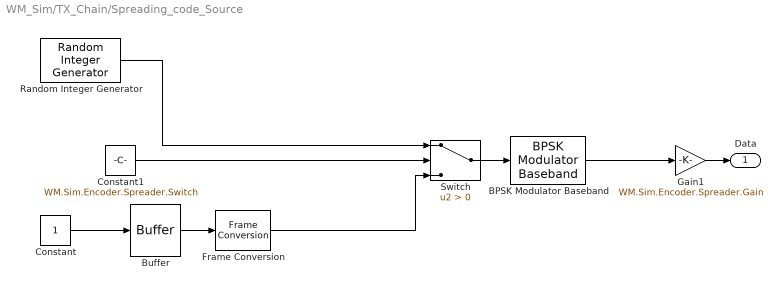
== system WM_Sim/TX_Chain/Spreading_code_Source ==
  BPSK Modulator Baseband : commdigbbndpm3/BPSK Modulator Baseband  Ph=0  outDtype=double  outWordLen=16  outUDDataType=sfix(16)  outFracLenMode=Best precision  outFracLen=15
  Buffer : Buffer  N=int32(WM.Sim.Frame_len)  TreatMby1Signals=One channel
  Constant : Constant  VectorParams1D=off  SampleTime=WM.Sim.SampleTimes.Tspreader  FramePeriod=WM.Sim.SampleTimes.Tspreader
      settings: SamplingMode=Frame based
  Constant1 : Constant  Value=WM.Sim.Encoder.Spreader.Switch  VectorParams1D=off  FramePeriod=WM.Sim.SampleTimes.Tspreader
  Frame Conversion : FrameConversion
  Gain1 : Gain  Gain=WM.Sim.Encoder.Spreader.Gain
  Random Integer Generator : commrandsrc2/Random Integer Generator  mul=WM.Sim.order_M  seed=WM.Sim.Encoder.Spreader.seed_code_real  Ts=WM.Sim.SampleTimes.Tspreader  frameBased=on  sampPerFrame=int32(WM.Sim.Frame_len)  orient=off  outDataType=double
  Switch : Switch  Criteria=u2 > Threshold
  Data : Outport
  wires:
  BPSK Modulator Baseband/1 -> Gain1/1
  Gain1/1 -> Data/1
  Constant/1 -> Buffer/1
  Random Integer Generator/1 -> Switch/1
  Switch/1 -> BPSK Modulator Baseband/1
  Constant1/1 -> Switch/2
  Buffer/1 -> Frame Conversion/1
  Frame Conversion/1 -> Switch/3

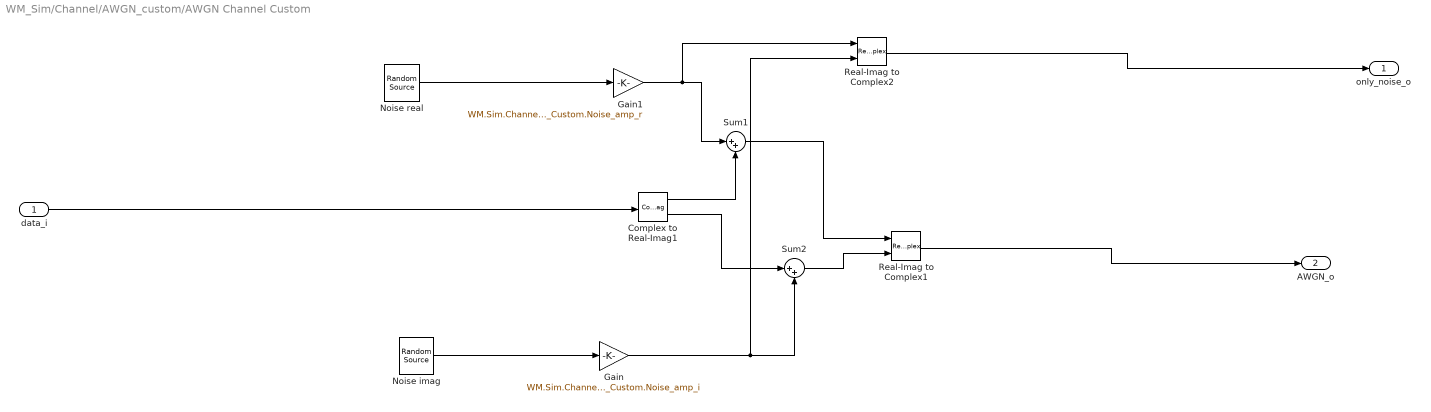
== system WM_Sim/Channel/AWGN_custom/AWGN Channel Custom ==
  data_i : Inport
  Complex to Real-Imag1 : ComplexToRealImag
  Gain : Gain  Gain=WM.Sim.Channel.AWGN_Custom.Noise_amp_i
  Gain1 : Gain  Gain=WM.Sim.Channel.AWGN_Custom.Noise_amp_r
  Noise imag : dspsrcs4/Random Source  SrcType=Gaussian  NormMethod=Ziggurat  CltLength=12  MinVal=0  MaxVal=1  MeanVal=0  VarVal=1  RepMode=Specify seed  rawSeed=WM.Sim.Channel.AWGN_Custom.seed_noise_imag  IsInherit=off  SampMode=Discrete  SampTime=WM.Sim.SampleTimes.Tchannel  SampFrame=int32(WM.Sim.Frame_len)  DataType=Double  OutComplex=Real
  Noise real : dspsrcs4/Random Source  SrcType=Gaussian  NormMethod=Ziggurat  CltLength=12  MinVal=0  MaxVal=1  MeanVal=0  VarVal=1  RepMode=Specify seed  rawSeed=WM.Sim.Channel.AWGN_Custom.seed_noise_real  IsInherit=off  SampMode=Discrete  SampTime=WM.Sim.SampleTimes.Tchannel  SampFrame=int32(WM.Sim.Frame_len)  DataType=Double  OutComplex=Real
  Real-Imag to Complex1 : RealImagToComplex
  Real-Imag to Complex2 : RealImagToComplex
  Sum1 : Sum  Inputs=|++
  Sum2 : Sum  Inputs=|++
  only_noise_o : Outport
  AWGN_o : Outport  Port=2
  wires:
  Complex to Real-Imag1/1 -> Sum1/2
  Complex to Real-Imag1/2 -> Sum2/1
  Real-Imag to Complex1/1 -> AWGN_o/1
  Real-Imag to Complex2/1 -> only_noise_o/1
  Sum1/1 -> Real-Imag to Complex1/1
  Noise imag/1 -> Gain/1
  Gain/1 -> Sum2/2, Real-Imag to Complex2/2
  Noise real/1 -> Gain1/1
  data_i/1 -> Complex to Real-Imag1/1
  Gain1/1 -> Sum1/1, Real-Imag to Complex2/1
  Sum2/1 -> Real-Imag to Complex1/2

== system WM_Sim/Channel/AWGN_custom/SNR_estimate ==
  out_block_i : Inport
  in_block_i : Inport  Port=2
  SNR_db1 : Display
  SNR_scope : Scope
      settings: YMin=-20.7608  YMax=-20.7587  SaveName=ScopeData4  MaxDataPoints=WM.Sim.SNR_Calc.Scope.Data_history_len
  Sum2 : Sum  Inputs=|-+
  custom awgn variance2 : dspstat3/Variance  run=on  reset_popup=None  InputProcessing=Columns as channels (frame based)  directionMode=Each column  dimension=1  treatSBRowAsCol=on  roiEnable=off  roiType=Rectangles  roiPortion=Entire ROI  roiOutput=Individual statistics for each ROI  roiFlag=off  roundingMode=Floor  overflowMode=off
  custom awgn variance3 : dspstat3/Variance  run=on  reset_popup=None  InputProcessing=Columns as channels (frame based)  directionMode=Each column  dimension=1  treatSBRowAsCol=on  roiEnable=off  roiType=Rectangles  roiPortion=Entire ROI  roiOutput=Individual statistics for each ROI  roiFlag=off  roundingMode=Floor  overflowMode=off
  dB Conversion2 : dspmathops/dB Conversion  dBtype=dB  intype=Power  R=1  fuzz=off
  dB Conversion3 : dspmathops/dB Conversion  dBtype=dB  intype=Power  R=1  fuzz=off
  wires:
  custom awgn variance2/1 -> dB Conversion3/1
  custom awgn variance3/1 -> dB Conversion2/1
  in_block_i/1 -> custom awgn variance2/1
  dB Conversion2/1 -> Sum2/1
  dB Conversion3/1 -> Sum2/2
  out_block_i/1 -> custom awgn variance3/1

== system WM_Sim/Channel/Audio_jammer/Audio_channel ==
  data_i : Inport
  Constant1 : Constant  Value=0  SampleTime=WM.Sim.Frame_len/WM.Sim.Fs_audio
  From Multimedia File : dspvision/From Multimedia File  inputFilename=./audio_test/Balmorhea - Days.wav  loop=on  numPlays=1  outputStreams=Audio only  videoDataType=single  audioDataType=double  inheritSampleTime=on  userDefinedSampleTime=1/30  noAudioOutput=off  isIntensityVideo=off  fourcc=RGB  colorVideoFormat=Separate color signals  outputEOF=off  dataOrg=Column-major  audioFrameSize=int32(WM.Sim.Frame_len)  computeAudioFrameSize=off  outSamplingMode=Frame based
  Real-Imag to Complex : RealImagToComplex
  Selector : Selector  NumberOfDimensions=2  InputPortWidth=2  IndexOptions=Select all,Index vector (dialog)  Indices=[1],1  OutputSizes=1,1
  Sum : Sum  Inputs=|++
  mix_o : Outport
  Jamm_o : Outport  Port=2
  wires:
  data_i/1 -> Sum/1
  Sum/1 -> mix_o/1
  From Multimedia File/1 -> Selector/1
  Selector/1 -> Real-Imag to Complex/1
  Constant1/1 -> Real-Imag to Complex/2
  Real-Imag to Complex/1 -> Jamm_o/1, Sum/2

== matlab function WM_Sim/RX_chain/Integrate and Dump Custom/Integrate and dumo ==
  data: u input; y output; WM parameter
function y = Idump(u,WM)
%#codegen

persistent data_on_hold
persistent offset
n_rows = size(u,1);
n_cols = size(u,2);

int_len = WM.Sim.Encoder.SF;
u_int  = complex(zeros(n_rows*n_cols,1));

effective_frame_len = (WM.Sim.Frame_len);

% if (real(u(1)) ~=0)
%     aa=1;
% end

for i=1:n_cols
    for j=1:n_rows
        u_int((j-1)*n_cols+i)=u(j,i);
    end
end


if isempty(data_on_hold)
    
    data_on_hold = complex(zeros(int_len,1));
    
end

if isempty(offset)
    if (effective_frame_len)==1
    
    offset = 0+ WM.Sim.IntDump.AddictionalOffset;
    
    else
         offset = mod(effective_frame_len+ WM.Sim.IntDump.AddictionalOffset,WM.Sim.Encoder.SF);
    
    end
    
end



if size(u,1)~=int_len
    
    error('column length must be equal to SF');    
end
len_data = length(u_int);
total_int_data = size(u,2)*int_len;
if offset==0
    n_SF_block_useful_current_frame=len_data/WM.Sim.Encoder.SF;
else
    n_SF_block_useful_current_frame = fix((len_data-double(offset))/WM.Sim.Encoder.SF);
end

%%%array init

data_2_int=complex(zeros(total_int_data,1));
data_2_int_2=complex(zeros(int_len,size(u,2)));






len_reminder = mod((len_data-offset),WM.Sim.Encoder.SF);

% if offset~=0 && len_reminder~=(int_len-offset)
%     
%     error('size problem');
%     
% end


%aggancio parte vecchia
if len_reminder>0
data_on_hold(:,1)=[data_on_hold(1:len_reminder);u_int(1:offset)];
end
last_useful_idx = offset+n_SF_block_useful_current_frame*WM.Sim.Encoder.SF;
data_useful_current_frame=u_int(offset+1:last_useful_idx);
if len_reminder>0
data_2_int(:,1) = [data_on_hold;data_useful_current_frame];
data_on_hold(1:len_reminder)=u_int(last_useful_idx+1:len_data);
offset = int_len-len_reminder;
else
    data_2_int(:,1) = data_useful_current_frame;
    offset = (0);
end




data_2_int_2(:,:) = reshape(data_2_int,int_len,n_cols);

y = sum(data_2_int_2,1);

end

== matlab function WM_Sim/SNR_ctrl/Pow_estimat/spect_pow_idx_calc ==
  data: spect input; freq input; out output; WM parameter
function out  = fcn(spect,freq,WM)
%#codegen


n_bins =size(spect,1);%% WM.Sim.Frame_len/WM.Sim.FEC_ratio;

fmax = WM.Sim.Fs_audio;

bin  = fmax/(n_bins-1);

% f_axe = 0 : bin : fmax;

left_freq = freq+WM.Sim.Encoder.Tx_BW;

right_freq = fmax+(freq-WM.Sim.Encoder.Tx_BW);

right_bin = ceil(right_freq/bin);
left_bin = fix(left_freq/bin);

% idx_array1 = ;
% idx_array2 =;

summa = sum(spect(1:left_bin))+sum(spect( right_bin:n_bins));

compones = 1/WM.Sim.Frame_len^2*summa;

out = repmat(compones,WM.Sim.Frame_len,1);
